simulink model "comparative_study"  (R2025b)
settings: Solver=VariableStepAuto  StartTime=0.0  StopTime=10.0  RelTol=1e-3
model workspace (MAT data in the model file):
  L = 2.65
  Lh = 0
  k = 1
  theta_d = 1
settings Model: Creator=yasin  LastModifiedBy=yasin

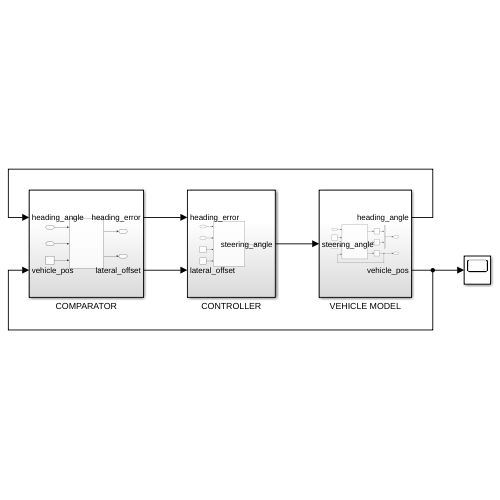
[thumbnail: Simulink's stored preview of the top-level diagram]
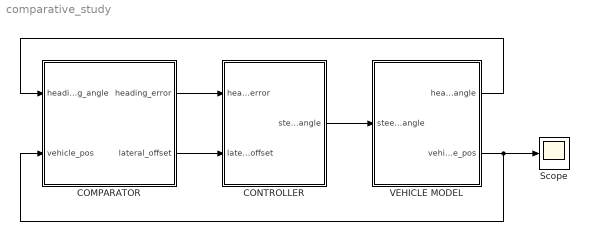
== system comparative_study ==
  COMPARATOR : Subsystem
  CONTROLLER : Subsystem
  Scope : Scope
      settings: ActiveDisplayYMinimum=-1  ActiveDisplayYMaximum=1
  VEHICLE MODEL : Subsystem
  wires:
  CONTROLLER/1(steering_angle) -> VEHICLE MODEL/1(steering_angle)
  COMPARATOR/1(heading_error) -> CONTROLLER/1(heading_error)
  COMPARATOR/2(lateral_offset) -> CONTROLLER/2(lateral_offset)
  VEHICLE MODEL/1(heading_angle) -> COMPARATOR/1(heading_angle)
  VEHICLE MODEL/2(vehicle_pos) -> COMPARATOR/2(vehicle_pos), Scope/1

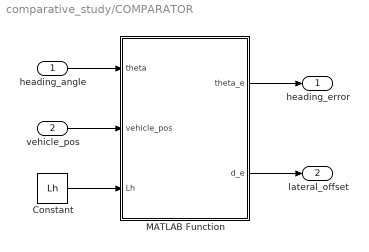
== system comparative_study/COMPARATOR ==
  heading_angle : Inport
  vehicle_pos : Inport  Port=2
  Constant : Constant  Value=Lh
  MATLAB Function : MATLAB Function  TreatAsAtomicUnit=on
  heading_error : Outport
  lateral_offset : Outport  Port=2
  wires:
  heading_angle/1 -> MATLAB Function/1(theta)
  vehicle_pos/1 -> MATLAB Function/2(vehicle_pos)
  MATLAB Function/1(theta_e) -> heading_error/1
  MATLAB Function/2(d_e) -> lateral_offset/1
  Constant/1 -> MATLAB Function/3(Lh)

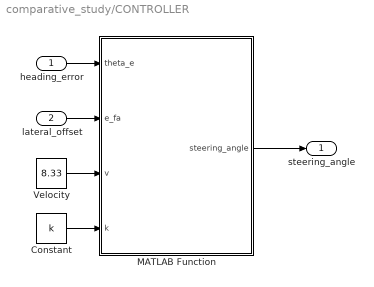
== system comparative_study/CONTROLLER ==
  heading_error : Inport
  lateral_offset : Inport  Port=2
  Constant : Constant  Value=k
  MATLAB Function : MATLAB Function  TreatAsAtomicUnit=on
  Velocity : Constant  Value=8.33
  steering_angle : Outport
  wires:
  heading_error/1 -> MATLAB Function/1(theta_e)
  lateral_offset/1 -> MATLAB Function/2(e_fa)
  MATLAB Function/1(steering_angle) -> steering_angle/1
  Velocity/1 -> MATLAB Function/3(v)
  Constant/1 -> MATLAB Function/4(k)

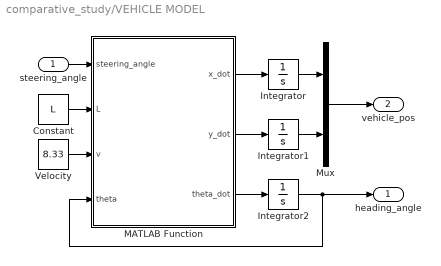
== system comparative_study/VEHICLE MODEL ==
  steering_angle : Inport
  Constant : Constant  Value=L
  Integrator : Integrator
  Integrator1 : Integrator
  Integrator2 : Integrator
  MATLAB Function : MATLAB Function  TreatAsAtomicUnit=on
  Mux : Mux  Inputs=2
  Velocity : Constant  Value=8.33
  heading_angle : Outport
  vehicle_pos : Outport  Port=2
  wires:
  steering_angle/1 -> MATLAB Function/1(steering_angle)
  Constant/1 -> MATLAB Function/2(L)
  MATLAB Function/1(x_dot) -> Integrator/1
  MATLAB Function/2(y_dot) -> Integrator1/1
  MATLAB Function/3(theta_dot) -> Integrator2/1
  Mux/1 -> vehicle_pos/1
  Integrator2/1 -> MATLAB Function/4(theta), heading_angle/1
  Integrator/1 -> Mux/1
  Integrator1/1 -> Mux/2
  Velocity/1 -> MATLAB Function/3(v)

== matlab function comparative_study/COMPARATOR/MATLAB Function ==
  data: theta input; theta_e output; vehicle_pos input; d_e output; Lh input
function [theta_e, d_e]= fcn(theta, vehicle_pos, Lh)

x   = vehicle_pos(1);
y   = vehicle_pos(2);

x_d = 0:1:100;
y_d = 20*sin(2*pi*x_d/80);

theta_d = atan((pi/2)*cos(2*pi*x/80));
theta_e = theta-theta_d;

d_e = (x+Lh*cos(theta)-x_d)*sin(theta_d) + (-y-Lh*sin(theta)+y_d)*cos(theta_d);

== matlab function comparative_study/VEHICLE MODEL/MATLAB Function ==
  data: steering_angle input; x_dot output; y_dot output; L input; v input; theta_dot output; theta input
function [x_dot, y_dot, theta_dot]  = fcn(steering_angle, L, v, theta)

x_dot     = v*cos(theta);
y_dot     = v*sin(theta);
theta_dot = v*tan(steering_angle)/L;

== matlab function comparative_study/CONTROLLER/MATLAB Function ==
  data: theta_e input; steering_angle output; e_fa input; v input; k input
function steering_angle = stanley(theta_e, e_fa, v, k)

steering_angle = theta_e + atan(k*e_fa/v);
